simulink model "Tekercs_K6_Alap"  (R2025a)
settings: Solver=VariableStepAuto  StartTime=0.0  StopTime=10e-3  MaxStep=1e-3/25  RelTol=1e-3
settings Model: Creator=Szalay  LastModifiedBy=Szalay

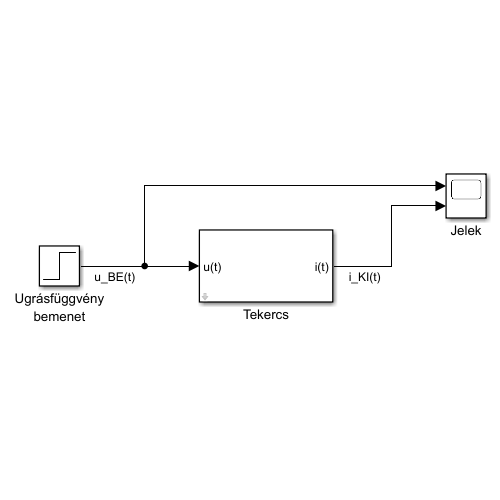
[thumbnail: Simulink's stored preview of the top-level diagram]
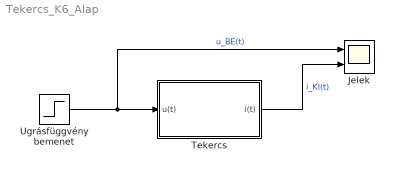
== system Tekercs_K6_Alap ==
  Jelek : Scope  NumInputPorts=2
      settings: ActiveDisplayYMinimum=-0.12499999999999997  ActiveDisplayYMaximum=1.125
  Tekercs : Subsystem  mask(Tekercs){L=2e-3, R=2, i_0=0.5}
      mask prompts: L "Öninduktivitás (H)"; R "Ellenállás (Ohm)"; i_0 "Kezdeti áramerősség (A)"
      mask help: Lineáris mágnesezettségű tekercs modell (RL-tag).
      mask DialogControl ParameterGroupVar Prompt: Modellparaméterek
      mask DialogControl Container3 Prompt: Kezdeti érték
  Ugrásfüggvény bemenet : Step  Time=5e-3  SampleTime=0
  wires:
  Ugrásfüggvény bemenet/1 -> Jelek/1, Tekercs/1(u(t))  "u_BE(t)"
  Tekercs/1(i(t)) -> Jelek/2  "i_KI(t)"

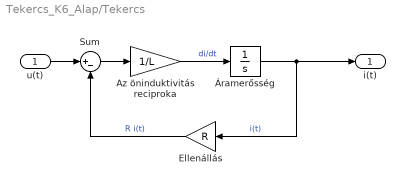
== system Tekercs_K6_Alap/Tekercs ==
  u(t) : Inport
  Az öninduktivitás reciproka : Gain  Gain=1/L
  Ellenállás : Gain  Gain=R
  Sum : Sum  Inputs=|+-
  Áramerősség : Integrator  InitialCondition=i_0
  i(t) : Outport
  wires:
  Áramerősség/1 -> i(t)/1, Ellenállás/1  "i(t)"
  Az öninduktivitás reciproka/1 -> Áramerősség/1  "di/dt"
  Ellenállás/1 -> Sum/2  "R i(t)"
  Sum/1 -> Az öninduktivitás reciproka/1
  u(t)/1 -> Sum/1
